simulink model "KLD"  (R2018a)
settings: Solver=VariableStepAuto  StartTime=0.0  StopTime=10.0  RelTol=1e-3
settings Model: Creator=aoki-soya  LastModifiedBy=aoki-soya

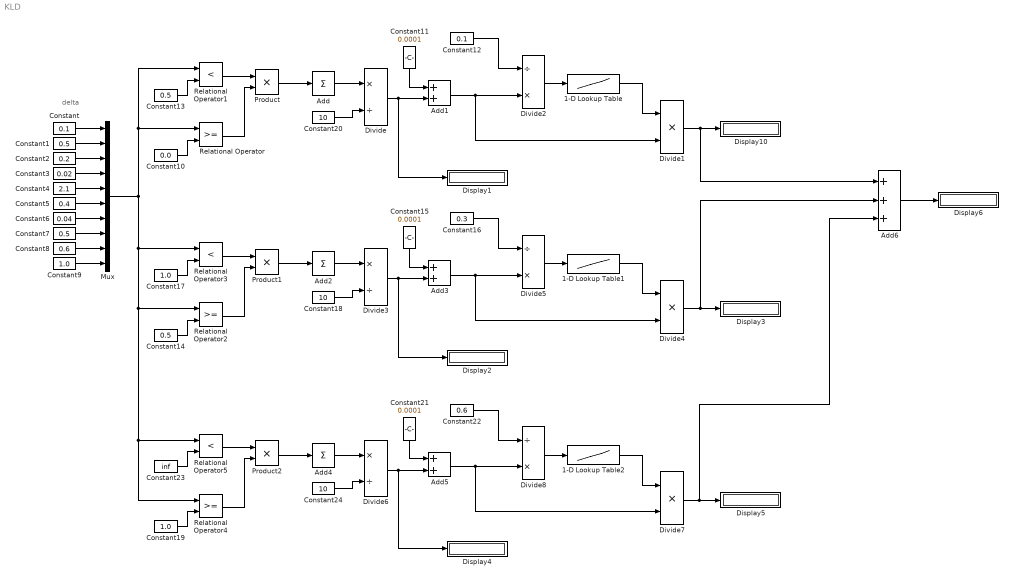
== system KLD ==
  note: delta
  1-D Lookup Table : Lookup_n-D  NumberOfTableDimensions=1  BreakpointsSpecification=Even spacing  BreakpointsForDimension1=[0:1]  BreakpointsForDimension1FirstPoint=0  BreakpointsForDimension1Spacing=0.1  Table=log([0:0.1:10])  InternalRulePriority=Speed  RndMeth=Simplest  InputSameDT=on
  1-D Lookup Table1 : Lookup_n-D  NumberOfTableDimensions=1  BreakpointsSpecification=Even spacing  BreakpointsForDimension1=[0:1]  BreakpointsForDimension1FirstPoint=0  BreakpointsForDimension1Spacing=0.1  Table=log([0:0.1:10])  InternalRulePriority=Speed  RndMeth=Simplest  InputSameDT=on
  1-D Lookup Table2 : Lookup_n-D  NumberOfTableDimensions=1  BreakpointsSpecification=Even spacing  BreakpointsForDimension1=[0:1]  BreakpointsForDimension1FirstPoint=0  BreakpointsForDimension1Spacing=0.1  Table=log([0:0.1:10])  InternalRulePriority=Speed  RndMeth=Simplest  InputSameDT=on
  Add : Sum  Inputs=+
  Add1 : Sum
  Add2 : Sum  Inputs=+
  Add3 : Sum
  Add4 : Sum  Inputs=+
  Add5 : Sum
  Add6 : Sum  Inputs=+++
  Constant : Constant  Value=0.1
  Constant{1,7,13..14} (4 alike) : Constant  Value=0.5
  Constant10 : Constant  Value=0.0
  Constant11 : Constant  Value=0.0001
  Constant12 : Constant  Value=0.1
  Constant15 : Constant  Value=0.0001
  Constant16 : Constant  Value=0.3
  Constant17 : Constant  Value=1.0
  Constant18 : Constant  Value=10
  Constant19 : Constant  Value=1.0
  Constant2 : Constant  Value=0.2
  Constant20 : Constant  Value=10
  Constant21 : Constant  Value=0.0001
  Constant22 : Constant  Value=0.6
  Constant23 : Constant  Value=inf
  Constant24 : Constant  Value=10
  Constant3 : Constant  Value=0.02
  Constant4 : Constant  Value=2.1
  Constant5 : Constant  Value=0.4
  Constant6 : Constant  Value=0.04
  Constant8 : Constant  Value=0.6
  Constant9 : Constant  Value=1.0
  Display{1..6,10} (7 alike) : Display
  Divide : Product  Inputs=*/
  Divide1 : Product  Inputs=**
  Divide2 : Product  Inputs=/*
  Divide3 : Product  Inputs=*/
  Divide4 : Product  Inputs=**
  Divide5 : Product  Inputs=/*
  Divide6 : Product  Inputs=*/
  Divide7 : Product  Inputs=**
  Divide8 : Product  Inputs=/*
  Mux : Mux  Inputs=10
  Product : Product
  Product1 : Product
  Product2 : Product
  Relational Operator : RelationalOperator  OutDataTypeStr=boolean  RndMeth=Simplest
  Relational Operator1 : RelationalOperator  Operator=<  OutDataTypeStr=boolean  RndMeth=Simplest
  Relational Operator2 : RelationalOperator  OutDataTypeStr=boolean  RndMeth=Simplest
  Relational Operator3 : RelationalOperator  Operator=<  OutDataTypeStr=boolean  RndMeth=Simplest
  Relational Operator4 : RelationalOperator  OutDataTypeStr=boolean  RndMeth=Simplest
  Relational Operator5 : RelationalOperator  Operator=<  OutDataTypeStr=boolean  RndMeth=Simplest
  wires:
  Constant7/1 -> Mux/8
  Constant/1 -> Mux/1
  Constant5/1 -> Mux/6
  Constant3/1 -> Mux/4
  Constant4/1 -> Mux/5
  Constant1/1 -> Mux/2
  Constant9/1 -> Mux/10
  Constant8/1 -> Mux/9
  Constant6/1 -> Mux/7
  Constant2/1 -> Mux/3
  Constant10/1 -> Relational Operator/2
  Constant20/1 -> Divide/2
  1-D Lookup Table/1 -> Divide1/1
  Divide1/1 -> Add6/1, Display10/1
  Constant11/1 -> Add1/1
  Add/1 -> Divide/1
  Divide/1 -> Display1/1, Add1/2
  Add1/1 -> Divide2/2, Divide1/2
  Constant12/1 -> Divide2/1
  Divide2/1 -> 1-D Lookup Table/1
  Constant13/1 -> Relational Operator1/2
  Relational Operator1/1 -> Product/1
  Relational Operator/1 -> Product/2
  Product/1 -> Add/1
  Constant18/1 -> Divide3/2
  Divide5/1 -> 1-D Lookup Table1/1
  Constant16/1 -> Divide5/1
  Constant15/1 -> Add3/1
  Add3/1 -> Divide5/2, Divide4/2
  Add2/1 -> Divide3/1
  Relational Operator3/1 -> Product1/1
  Divide4/1 -> Add6/2, Display3/1
  Product1/1 -> Add2/1
  Divide3/1 -> Display2/1, Add3/2
  Relational Operator2/1 -> Product1/2
  Constant14/1 -> Relational Operator2/2
  Constant17/1 -> Relational Operator3/2
  1-D Lookup Table1/1 -> Divide4/1
  Divide8/1 -> 1-D Lookup Table2/1
  Constant19/1 -> Relational Operator4/2
  Relational Operator4/1 -> Product2/2
  Constant24/1 -> Divide6/2
  Add5/1 -> Divide8/2, Divide7/2
  Divide7/1 -> Add6/3, Display5/1
  Constant21/1 -> Add5/1
  1-D Lookup Table2/1 -> Divide7/1
  Add4/1 -> Divide6/1
  Relational Operator5/1 -> Product2/1
  Divide6/1 -> Display4/1, Add5/2
  Constant22/1 -> Divide8/1
  Mux/1 -> Relational Operator1/1, Relational Operator/1, Relational Operator4/1, Relational Operator5/1, Relational Operator2/1, Relational Operator3/1
  Constant23/1 -> Relational Operator5/2
  Product2/1 -> Add4/1
  Add6/1 -> Display6/1
